simulink model "Lab8_2"  (R2019a)
settings: Solver=ode45  StartTime=0.0  StopTime=0.5  RelTol=1e-3
libraries: commutil2 x2, commsrccod2 x2
settings Model: Creator=ouoam  LastModifiedBy=ouoam

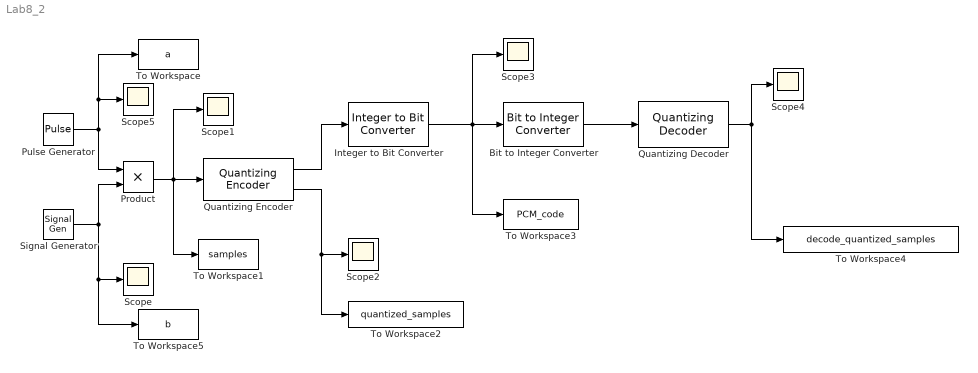
== system Lab8_2 ==
  Bit to Integer Converter : commutil2/Bit to Integer Converter  nbits=3  bitOrder=MSB first  signedOutputValues=Unsigned  outDtype=Inherit via internal rule  outDtypeSigned=Inherit via internal rule
      settings: SourceProductName=Communications Toolbox
  Integer to Bit Converter : commutil2/Integer to Bit Converter  nbits=3  signedInputValues=Unsigned  bitOrder=MSB first  outDtype=Inherit via internal rule
      settings: SourceProductName=Communications Toolbox
  Product : Product
  Pulse Generator : DiscretePulseGenerator  PulseType=Time based  Period=0.01
  Quantizing Decoder : commsrccod2/Quantizing Decoder  codebook=[-1.75 -1.25 -.75 -.25 .25 .75 1.25 1.75]  QuDType=double
      settings: SourceProductName=Communications Toolbox  SourceProductBaseCode=CM
  Quantizing Encoder : commsrccod2/Quantizing Encoder  partition=[-1.5 -1 -.5 0 .5 1 1.5]  codebook=[-1.75 -1.25 -.75 -.25 .25 .75 1.25 1.75]  idxDType=double
      settings: SourceProductName=Communications Toolbox  SourceProductBaseCode=CM
  Scope{,1..5} (6 alike) : Scope
  Signal Generator : SignalGenerator  Amplitude=2  Frequency=5
  To Workspace : ToWorkspace  VariableName=a  SaveFormat=Timeseries  SampleTime=-1
  To Workspace1 : ToWorkspace  VariableName=samples  SampleTime=0.01
  To Workspace2 : ToWorkspace  VariableName=quantized_samples  SampleTime=0.01
  To Workspace3 : ToWorkspace  VariableName=PCM_code  SampleTime=0.01
  To Workspace4 : ToWorkspace  VariableName=decode_quantized_samples  SampleTime=0.01
  To Workspace5 : ToWorkspace  VariableName=b  SaveFormat=Timeseries  SampleTime=-1
  wires:
  Pulse Generator/1 -> To Workspace/1, Scope5/1, Product/1
  Signal Generator/1 -> Product/2, To Workspace5/1, Scope/1
  Product/1 -> Quantizing Encoder/1, To Workspace1/1, Scope1/1
  Integer to Bit Converter/1 -> To Workspace3/1, Scope3/1, Bit to Integer Converter/1
  Bit to Integer Converter/1 -> Quantizing Decoder/1
  Quantizing Decoder/1 -> To Workspace4/1, Scope4/1
  Quantizing Encoder/1 -> Integer to Bit Converter/1
  Quantizing Encoder/2 -> To Workspace2/1, Scope2/1
